simulink model "chap1_5"  (R2016a)
settings: Solver=ode45  StartTime=0.0  StopTime=10.0  RelTol=1e-3
settings Model: Creator=zhanghankui  LastModifiedBy=zhanghankui

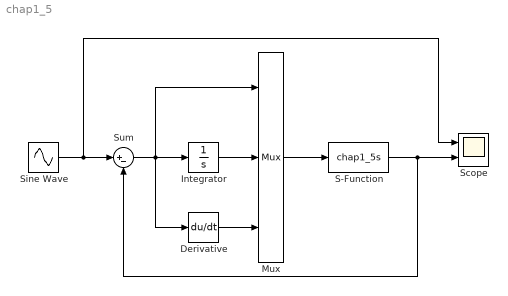
== system chap1_5 ==
  Derivative : Derivative
  Integrator : Integrator
  Mux : Mux  Inputs=3
  S-Function : S-Function  FunctionName=chap1_5s  SFunctionDeploymentMode=off  EnableBusSupport=off
  Scope : Scope  NumInputPorts=2
  Sine Wave : Sin  Amplitude=0.5  Frequency=2*pi  SampleTime=0
  Sum : Sum  Inputs=|+-
  wires:
  Sine Wave/1 -> Scope/1, Sum/1
  Sum/1 -> Mux/1, Derivative/1, Integrator/1
  Derivative/1 -> Mux/3
  Integrator/1 -> Mux/2
  Mux/1 -> S-Function/1
  S-Function/1 -> Scope/2, Sum/2
